simulink library "Plant"  (Simulink 7.8)
settings: Solver=ode45  StartTime=0.0  StopTime=10.0  RelTol=1e-3
undefined symbols (not defined in the file): beaver_b, beaver_c, beaver_init_p, beaver_init_pitch, beaver_init_q, beaver_init_r, beaver_init_roll, beaver_mass, Cl0, Cl_alpha2_dpt, Cl_beta, Cl_da, Cl_da_alpha, Cl_dr, Cl_p, Cl_r, Cm0, Cm_alpha, Cm_alpha2, Cm_beta2, Cm_de, Cm_df, Cm_dpt, Cm_q, Cm_r, Cn0, Cn_beta, Cn_beta3, Cn_da, Cn_dpt3, Cn_dr, Cn_p, Cn_q, Cn_r, Cx0, Cx_alpha, Cx_alpha2, Cx_alpha3, Cx_df, Cx_df_alpha, Cx_dpt, Cx_dpt2_alpha, Cx_dr, Cx_q, Cy0, Cy_beta, Cy_da, Cy_dr, Cy_dr_alpha, Cy_p, Cy_r, Cz0, Cz_alpha, Cz_alpha3, Cz_de, Cz_de_beta, Cz_df, Cz_df_alpha, Cz_dpt, Cz_q ... (+8)
libraries: aerolibconvert2 x5, aerolibasang x3, aerolibactuator x3, aerolibwind2 x3, aerolib6dof2 x1, aerolibadyn x1, aerolibatmos2 x1, aerolibobsolete x1, simulink x1
settings Model: Creator=fguerin  LastModifiedBy=fguerin

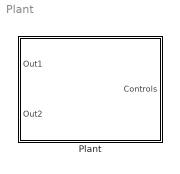
== system Plant ==
  Plant : Subsystem  TreatAsAtomicUnit=on
      mask Display: image(imread('asbbeaver.jpg'))

== system Plant/Plant ==
  Controls : Inport
  Air Data Sensor : Subsystem  TreatAsAtomicUnit=on
  DeHavilland Beaver Airframe : Subsystem
  Environment : Subsystem
  Inertial Data Sensor : Subsystem  TreatAsAtomicUnit=on
  Model Info : simulink/Model-Wide Utilities/Model Info  InitialBlockCM=None  BlockCM=None  Frame=on  DisplayStringWithTags=|  HorizontalTextAlignment=Center  LeftAlignmentValue=0.5  SourceBlockDiagram=Plant  TagMaxNumber=20
      | DeHavilland Beaver model 
      | based on original work created by
      | Marc Rauw for Delft University of Technology.  
      | http://www.dutchroll.com
  Out1 : Outport
  Out2 : Outport  Port=2
  wires:
  Controls/1 -> DeHavilland Beaver Airframe/2(Pilot)
  Air Data Sensor/1(Air Data) -> Out2/1
  Inertial Data Sensor/1(Inertial) -> Out1/1
  Environment/1(EnvBus) -> DeHavilland Beaver Airframe/1(EnvirBus)
  DeHavilland Beaver Airframe/1(ACBus) -> Environment/1(ACBus), Air Data Sensor/1(AC Bus), Inertial Data Sensor/1(AC Bus)

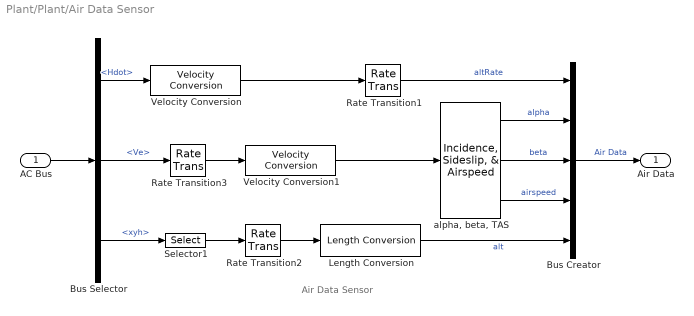
== system Plant/Plant/Air Data Sensor ==
  note: Air Data Sensor
  AC Bus : Inport
  Bus Creator : BusCreator  Inputs=5
  Bus Selector : BusSelector  OutputSignals=Hdot,Ve,xyh
  Length Conversion : aerolibconvert2/Length Conversion  IU=m  OU=ft
  Rate Transition1 : RateTransition  OutPortSampleTime=1/40
  Rate Transition2 : RateTransition  X0=2202  OutPortSampleTime=1/40
  Rate Transition3 : RateTransition  X0=[44.54 2.714 5.836]  OutPortSampleTime=1/40
  Selector1 : Selector  InputPortWidth=3  IndexOptions=Index vector (dialog)  Indices=[3]  OutputSizes=1
  Velocity Conversion : aerolibconvert2/Velocity Conversion  IU=m/s  OU=ft/s
  Velocity Conversion1 : aerolibconvert2/Velocity Conversion  IU=m/s  OU=ft/s
  "alpha, beta, TAS" : aerolibasang/Incidence, Sideslip, & Airspeed
  Air Data : Outport
  wires:
  Rate Transition2/1 -> Length Conversion/1
  Rate Transition3/1 -> Velocity Conversion1/1
  Velocity Conversion1/1 -> "alpha, beta, TAS"/1
  Length Conversion/1 -> Bus Creator/5  "alt"
  Velocity Conversion/1 -> Rate Transition1/1
  "alpha, beta, TAS"/3 -> Bus Creator/4  "airspeed"
  "alpha, beta, TAS"/2 -> Bus Creator/3  "beta"
  "alpha, beta, TAS"/1 -> Bus Creator/2  "alpha"
  Selector1/1 -> Rate Transition2/1
  Rate Transition1/1 -> Bus Creator/1  "altRate"
  Bus Creator/1 -> Air Data/1  "Air Data"
  Bus Selector/3 -> Selector1/1  "<xyh>"
  Bus Selector/2 -> Rate Transition3/1  "<Ve>"
  Bus Selector/1 -> Velocity Conversion/1  "<Hdot>"
  AC Bus/1 -> Bus Selector/1

== system Plant/Plant/DeHavilland Beaver Airframe ==
  note: DeHavilland Beaver Airframe
  EnvirBus : Inport
  Pilot : Inport  Port=2
  Aircraft Dynamics : Subsystem
  Calculate Parameters : Subsystem
  ACBus : Outport
  wires:
  Calculate Parameters/1(FltParams) -> Aircraft Dynamics/3(FltParams)
  EnvirBus/1 -> Calculate Parameters/1(EnvirBus), Aircraft Dynamics/2(EnvirBus)
  Aircraft Dynamics/1(AC Bus) -> Calculate Parameters/2(ACBus), ACBus/1
  Pilot/1 -> Aircraft Dynamics/1(Pilot)

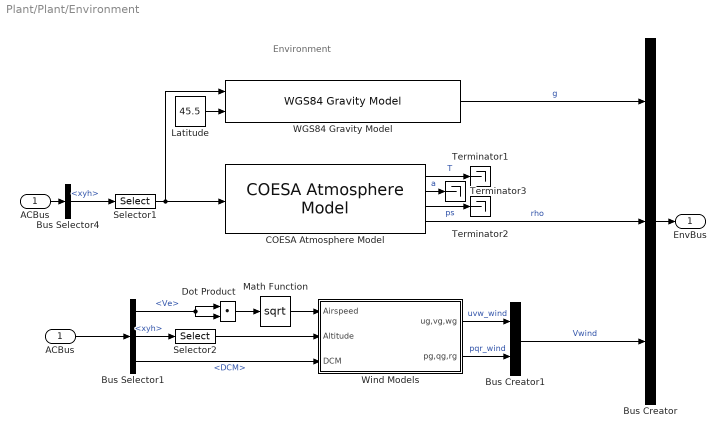
== system Plant/Plant/Environment ==
  note: Environment
  ACBus : Inport
  "ACBus " : InportShadow  Port=1
  Bus Creator : BusCreator  Inputs=3
  Bus Creator1 : BusCreator  Inputs=2
  Bus Selector1 : BusSelector  OutputSignals=Ve,xyh,DCM
  Bus Selector4 : BusSelector  OutputSignals=xyh
  COESA Atmosphere Model : aerolibatmos2/COESA Atmosphere Model  units=Metric (MKS)  spec=1976 COESA-extended U.S. Standard Atmosphere  model=Profile  profile_var=High temperature  profile_percent=1%  profile_alt=5 km (16404 ft)  envelope_var=High temperature  envelope_percent=1%  action=Warning
  Dot Product : DotProduct  InputSameDT=on  OutDataTypeStr=Inherit: Inherit via internal rule
  Latitude : Constant  Value=45.5
  Math Function : Math  Operator=sqrt  SaturateOnIntegerOverflow=on
  Selector1 : Selector  InputPortWidth=3  IndexOptions=Index vector (dialog)  Indices=[3]  OutputSizes=1
  Selector2 : Selector  InputPortWidth=3  IndexOptions=Index vector (dialog)  Indices=[3]  OutputSizes=1
  Terminator1 : Terminator
  Terminator2 : Terminator
  Terminator3 : Terminator
  WGS84 Gravity Model : aerolibobsolete/WGS84 Gravity Model  model=WGS84 Taylor Series  units=Metric (MKS)  no_atmos=on  precessing=on  month=February  day=1  year=2000  no_centrifugal=on  action=Warning
  Wind Models : Subsystem
  EnvBus : Outport
  wires:
  Bus Selector1/1 -> Dot Product/2, Dot Product/1  "<Ve>"
  Selector2/1 -> Wind Models/2(Altitude)
  Bus Selector1/2 -> Selector2/1  "<xyh>"
  "ACBus "/1 -> Bus Selector1/1
  Bus Selector4/1 -> Selector1/1  "<xyh>"
  ACBus/1 -> Bus Selector4/1
  Bus Creator/1 -> EnvBus/1
  Math Function/1 -> Wind Models/1(Airspeed)
  Dot Product/1 -> Math Function/1
  Bus Creator1/1 -> Bus Creator/3  "Vwind"
  Wind Models/1(ug,vg,wg) -> Bus Creator1/1  "uvw_wind"
  Wind Models/2(pg,qg,rg) -> Bus Creator1/2  "pqr_wind"
  Bus Selector1/3 -> Wind Models/3(DCM)  "<DCM>"
  WGS84 Gravity Model/1 -> Bus Creator/1  "g"
  Latitude/1 -> WGS84 Gravity Model/2
  Selector1/1 -> WGS84 Gravity Model/1, COESA Atmosphere Model/1
  COESA Atmosphere Model/2 -> Terminator3/1  "a"
  COESA Atmosphere Model/3 -> Terminator2/1  "ps"
  COESA Atmosphere Model/1 -> Terminator1/1  "T"
  COESA Atmosphere Model/4 -> Bus Creator/2  "rho"

== system Plant/Plant/Inertial Data Sensor ==
  note: Inertial Data Sensor
  AC Bus : Inport
  Angle Conversion3 : aerolibconvert2/Angle Conversion  IU=rad  OU=deg
  Angle Conversion5 : aerolibconvert2/Angle Conversion  IU=rad  OU=deg
  Bus Creator : BusCreator  Inputs=6
  Bus Selector : BusSelector  OutputSignals=phi_theta_psi,pqr
  Demux : Demux  Outputs=3
  Demux1 : Demux  Outputs=3
  Rate Transition1 : RateTransition  X0=beaver_init_roll/pi*180  OutPortSampleTime=1/40
  Rate Transition2 : RateTransition  X0=beaver_init_pitch/pi*180  OutPortSampleTime=1/40
  Rate Transition3 : RateTransition  X0=heading0  OutPortSampleTime=1/40
  Rate Transition4 : RateTransition  OutPortSampleTime=1/40
  Inertial : Outport
  wires:
  Angle Conversion5/1 -> Demux1/1
  Demux1/3 -> Rate Transition3/1
  Demux1/2 -> Rate Transition2/1
  Demux1/1 -> Rate Transition1/1
  Bus Selector/1 -> Angle Conversion5/1  "<phi_theta_psi>"
  Angle Conversion3/1 -> Rate Transition4/1
  Rate Transition4/1 -> Demux/1
  Rate Transition3/1 -> Bus Creator/3  "psi"
  Rate Transition2/1 -> Bus Creator/2  "theta"
  Rate Transition1/1 -> Bus Creator/1  "phi"
  Demux/1 -> Bus Creator/4  "p"
  Demux/3 -> Bus Creator/6  "r"
  Bus Creator/1 -> Inertial/1  "Inertial"
  Demux/2 -> Bus Creator/5  "q"
  Bus Selector/2 -> Angle Conversion3/1  "<pqr>"
  AC Bus/1 -> Bus Selector/1

== system Plant/Plant/DeHavilland Beaver Airframe/Aircraft Dynamics ==
  Pilot : Inport
  EnvirBus : Inport  Port=2
  FltParams : Inport  Port=3
  6DoF (Quaternion) : aerolib6dof2/6DoF (Euler Angles)  units=Metric (MKS)  mtype=Fixed  rep=Quaternion  xme_0=xme_0  Vm_0=[44.54 2.714 5.836]  eul_0=[beaver_init_roll, beaver_init_pitch, heading0/180*pi]  pm_0=[beaver_init_p, beaver_init_q, beaver_init_r]  mass_0=beaver_mass  mass_e=0  mass_f=0  inertia="[5.787969e3  0 1.1764e2; 0 6.92893e3 0; -1.1764e2 0 1.1578329e4]"  inertia_e=eye(3)  inertia_f=eye(3)  k_quat=1.0
  Bus Creator : BusCreator  Inputs=8
  Hdot : Gain  Gain=-1  SaturateOnIntegerOverflow=on  OutDataTypeStr=Inherit: Same as input  ParamDataTypeStr=Inherit: Same as input
  Selector1 : Selector  InputPortWidth=3  IndexOptions=Index vector (dialog)  Indices=[3]  OutputSizes=1
  Terminator : Terminator
  Terminator1 : Terminator
  Total Forces  and Moments : Subsystem
  xyH : Gain  Gain=[1 1 -1]  SaturateOnIntegerOverflow=on  OutDataTypeStr=Inherit: Same as input  ParamDataTypeStr=Inherit: Same as input
  AC Bus : Outport
  wires:
  FltParams/1 -> Total Forces  and Moments/4(FltParams)
  6DoF (Quaternion)/6 -> Bus Creator/8  "pqr"
  EnvirBus/1 -> Total Forces  and Moments/1(EnvirBus)
  Bus Creator/1 -> AC Bus/1
  6DoF (Quaternion)/8 -> Terminator1/1
  Hdot/1 -> Bus Creator/1  "Hdot"
  xyH/1 -> Bus Creator/4  "xyh"
  Total Forces  and Moments/2(Total Moment) -> 6DoF (Quaternion)/2
  Total Forces  and Moments/1(Total Force) -> 6DoF (Quaternion)/1
  Selector1/1 -> Hdot/1
  Pilot/1 -> Total Forces  and Moments/2(Pilot)
  6DoF (Quaternion)/1 -> Bus Creator/2, Selector1/1  "Ve"
  6DoF (Quaternion)/7 -> Terminator/1
  6DoF (Quaternion)/5 -> Bus Creator/7  "Vbody"
  6DoF (Quaternion)/2 -> Bus Creator/3, xyH/1  "Xe"
  6DoF (Quaternion)/3 -> Bus Creator/5  "phi_theta_psi"
  6DoF (Quaternion)/4 -> Total Forces  and Moments/3(DCM), Bus Creator/6  "DCM"

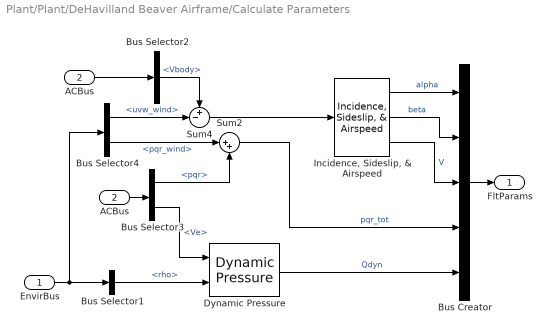
== system Plant/Plant/DeHavilland Beaver Airframe/Calculate Parameters ==
  EnvirBus : Inport
  ACBus : Inport  Port=2
  "ACBus " : InportShadow  Port=2
  Bus Creator : BusCreator  Inputs=5
  Bus Selector1 : BusSelector  OutputSignals=rho
  Bus Selector2 : BusSelector  OutputSignals=Vbody
  Bus Selector3 : BusSelector  OutputSignals=pqr,Ve
  Bus Selector4 : BusSelector  OutputSignals=Vwind.uvw_wind,Vwind.pqr_wind
  Dynamic Pressure : aerolibasang/Dynamic Pressure
  "Incidence, Sideslip, & Airspeed" : aerolibasang/Incidence, Sideslip, & Airspeed
  Sum2 : Sum  Inputs=|++  SaturateOnIntegerOverflow=on  InputSameDT=on  OutDataTypeStr=Inherit: Same as first input
  Sum4 : Sum  Inputs=+-|  SaturateOnIntegerOverflow=on  InputSameDT=on  OutDataTypeStr=Inherit: Same as first input
  FltParams : Outport
  wires:
  Sum2/1 -> Bus Creator/4  "pqr_tot"
  Bus Selector4/1 -> Sum4/2  "<uvw_wind>"
  Bus Selector2/1 -> Sum4/1  "<Vbody>"
  "Incidence, Sideslip, & Airspeed"/3 -> Bus Creator/3  "V"
  "Incidence, Sideslip, & Airspeed"/2 -> Bus Creator/2  "beta"
  "Incidence, Sideslip, & Airspeed"/1 -> Bus Creator/1  "alpha"
  Sum4/1 -> "Incidence, Sideslip, & Airspeed"/1
  Bus Selector4/2 -> Sum2/1  "<pqr_wind>"
  Bus Selector3/2 -> Dynamic Pressure/1  "<Ve>"
  Dynamic Pressure/1 -> Bus Creator/5  "Qdyn"
  EnvirBus/1 -> Bus Selector4/1, Bus Selector1/1
  Bus Selector1/1 -> Dynamic Pressure/2  "<rho>"
  ACBus/1 -> Bus Selector3/1
  Bus Selector3/1 -> Sum2/2  "<pqr>"
  Bus Creator/1 -> FltParams/1
  "ACBus "/1 -> Bus Selector2/1

== system Plant/Plant/Environment/Wind Models ==
  Airspeed : Inport
  Altitude : Inport  Port=2
  DCM : Inport  Port=3
  "DCM " : InportShadow  Port=3
  Discrete Wind Gust Model : aerolibwind2/Discrete Wind Gust Model  units=Metric (MKS)  Gx=off  Gy=off  Gz=off  t_0=20  d_m=[120 120 80]  v_m=[3.5 3.5 3.0]
  Dryden Wind Turbulence Model  (Continuous (+q -r)) : aerolibwind2/Dryden Wind Turbulence Model  (Continuous (+q -r))  units=Metric (MKS)  spec=MIL-F-8785C  model=Continuous Dryden (+q -r)  W20=5  Wdeg=0  TurbProb=10^-2 - Light  L_high=533.4  Wingspan=4  ts=0.1  Seed=[23341 23342 23343 23344]  T_on=off
  Sum : Sum  Inputs=+++  SaturateOnIntegerOverflow=on  InputSameDT=on  OutDataTypeStr=Inherit: Same as first input
  Wind Shear Model : aerolibwind2/Wind Shear Model  units=Metric (MKS)  phase=Category C - Terminal Flight Phase  W_20=0  Wdeg=0
  ug,vg,wg : Outport
  pg,qg,rg : Outport  Port=2
  wires:
  Altitude/1 -> Wind Shear Model/1, Dryden Wind Turbulence Model  (Continuous (+q -r))/1
  Dryden Wind Turbulence Model  (Continuous (+q -r))/2 -> pg,qg,rg/1
  Airspeed/1 -> Discrete Wind Gust Model/1, Dryden Wind Turbulence Model  (Continuous (+q -r))/2
  DCM/1 -> Wind Shear Model/2
  Sum/1 -> ug,vg,wg/1
  Discrete Wind Gust Model/1 -> Sum/3
  Dryden Wind Turbulence Model  (Continuous (+q -r))/1 -> Sum/2
  Wind Shear Model/1 -> Sum/1
  "DCM "/1 -> Dryden Wind Turbulence Model  (Continuous (+q -r))/3

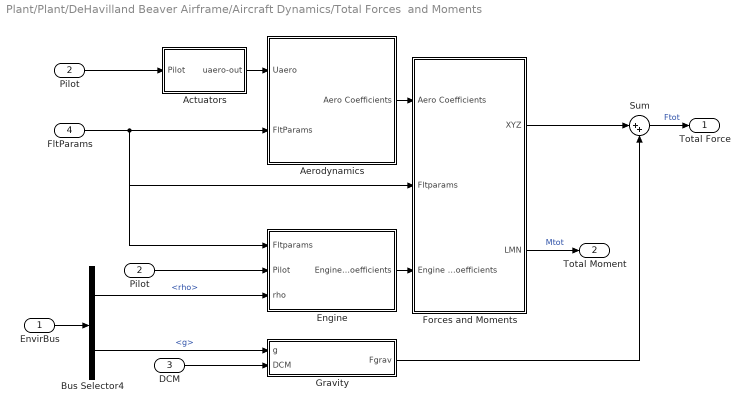
== system Plant/Plant/DeHavilland Beaver Airframe/Aircraft Dynamics/Total Forces  and Moments ==
  EnvirBus : Inport
  Pilot : Inport  Port=2
  DCM : Inport  Port=3
  FltParams : Inport  Port=4
  Actuators : Subsystem
  Aerodynamics : Subsystem
  Bus Selector4 : BusSelector  OutputSignals=rho,g
  "Engine " : Subsystem
  Forces and Moments : Subsystem
  "Gravity " : Subsystem
  "Pilot " : InportShadow  Port=2
  Sum : Sum  Inputs=|++  SaturateOnIntegerOverflow=on  InputSameDT=on  OutDataTypeStr=Inherit: Same as first input
  Total Force : Outport
  Total Moment : Outport  Port=2
  wires:
  EnvirBus/1 -> Bus Selector4/1
  Actuators/1(uaero-out) -> Aerodynamics/1(Uaero)
  FltParams/1 -> Aerodynamics/2(FltParams), Forces and Moments/2(Fltparams), "Engine "/1(Fltparams)
  "Pilot "/1 -> "Engine "/2(Pilot)
  Forces and Moments/2(LMN) -> Total Moment/1  "Mtot"
  Sum/1 -> Total Force/1  "Ftot"
  Bus Selector4/2 -> "Gravity "/1(g)  "<g>"
  DCM/1 -> "Gravity "/2(DCM)
  Bus Selector4/1 -> "Engine "/3(rho)  "<rho>"
  Pilot/1 -> Actuators/1(Pilot)
  Aerodynamics/1(Aero Coefficients) -> Forces and Moments/1(Aero Coefficients)
  "Gravity "/1(Fgrav) -> Sum/2
  "Engine "/1(Engine Coefficients) -> Forces and Moments/3(Engine Coefficients)
  Forces and Moments/1(XYZ) -> Sum/1

== system Plant/Plant/DeHavilland Beaver Airframe/Aircraft Dynamics/Total Forces  and Moments/Actuators ==
  Pilot : Inport
  Aileron Actuator : aerolibactuator/Second Order Nonlinear Actuator  wn_fin=10*2*pi  z_fin=0.7  fin_max=15*pi/180  fin_min=-15*pi/180  fin_maxrate=40*pi/180  fin_act_0=uaero0(3)
  Bus Selector2 : BusSelector  OutputSignals=uaero
  Demux : Demux
  Elevator Actuator : aerolibactuator/Second Order Nonlinear Actuator  wn_fin=10*2*pi  z_fin=0.7  fin_max=20*pi/180  fin_min=-20*pi/180  fin_maxrate=40*pi/180  fin_act_0=uaero0(1)
  Initial inputs for aero : Constant  Value=uaero0
  Mux : Mux
  Rudder Actuator : aerolibactuator/Second Order Nonlinear Actuator  wn_fin=10*2*pi  z_fin=0.7  fin_max=25*pi/180  fin_min=-25*pi/180  fin_maxrate=40*pi/180  fin_act_0=uaero0(3)
  Sum1 : Sum  Inputs=++|  SaturateOnIntegerOverflow=on  InputSameDT=on  OutDataTypeStr=Inherit: Same as first input
  uaero-out : Outport
  wires:
  Rudder Actuator/1 -> Mux/3
  Aileron Actuator/1 -> Mux/2
  Elevator Actuator/1 -> Mux/1
  Bus Selector2/1 -> Sum1/2  "<uaero>"
  Sum1/1 -> Demux/1
  Mux/1 -> uaero-out/1
  Demux/3 -> Rudder Actuator/1
  Demux/2 -> Aileron Actuator/1
  Demux/1 -> Elevator Actuator/1
  Demux/4 -> Mux/4
  Initial inputs for aero/1 -> Sum1/1
  Pilot/1 -> Bus Selector2/1

== system Plant/Plant/DeHavilland Beaver Airframe/Aircraft Dynamics/Total Forces  and Moments/Aerodynamics ==
  Uaero : Inport
  FltParams : Inport  Port=2
  Actuator Increments : Subsystem
  Body Rate Damping : Subsystem
  Bus Selector1 : BusSelector  OutputSignals=alpha,beta
  Bus Selector2 : BusSelector  OutputSignals=V,pqr_tot
  Datum Coefficients : Subsystem
  Sum : Sum  Inputs=+++  SaturateOnIntegerOverflow=on
  Aero Coefficients : Outport
  wires:
  FltParams/1 -> Bus Selector2/1, Bus Selector1/1
  Bus Selector1/1 -> Datum Coefficients/1(alpha), Actuator Increments/1(alpha)  "<alpha>"
  Uaero/1 -> Actuator Increments/3(Actuator Deflections)
  Bus Selector2/2 -> Body Rate Damping/2(p,q,r)  "<pqr_tot>"
  Bus Selector2/1 -> Body Rate Damping/1(V)  "<V>"
  Actuator Increments/1(Coefficients) -> Sum/2
  Datum Coefficients/1(Coefficients) -> Sum/1
  Body Rate Damping/1(Coefficients) -> Sum/3
  Sum/1 -> Aero Coefficients/1
  Bus Selector1/2 -> Datum Coefficients/2(beta), Actuator Increments/2(beta)  "<beta>"

== system Plant/Plant/DeHavilland Beaver Airframe/Aircraft Dynamics/Total Forces  and Moments/Engine  ==
  Fltparams : Inport
  Pilot : Inport  Port=2
  rho : Inport  Port=3
  Bus Selector4 : BusSelector  OutputSignals=V,alpha
  eng : Subsystem
  pow : Subsystem
  Engine Coefficients : Outport
  wires:
  Fltparams/1 -> Bus Selector4/1
  pow/1(dpt) -> eng/1(dpt)
  Pilot/1 -> pow/2(Pilot)
  eng/1(Cprop) -> Engine Coefficients/1
  Bus Selector4/2 -> eng/2(alpha)  "<alpha>"
  rho/1 -> pow/1(rho)
  Bus Selector4/1 -> pow/3(V)  "<V>"

== system Plant/Plant/DeHavilland Beaver Airframe/Aircraft Dynamics/Total Forces  and Moments/Forces and Moments ==
  Aero Coefficients : Inport
  Fltparams : Inport  Port=2
  Engine Coefficients : Inport  Port=3
  Aerodynamic Forces and Moments : aerolibadyn/Aerodynamic Forces and Moments   inputAxes=Body  outputForceAxes=Body  outputMomentAxes=Body  S=beaver_S  b=beaver_b  cbar=beaver_c
  Bus Selector4 : BusSelector  OutputSignals=Qdyn
  Sum : Sum  Inputs=++|  SaturateOnIntegerOverflow=on  InputSameDT=on  OutDataTypeStr=Inherit: Same as first input
  neglect center of gravity  and center of pressure effects : Constant  Value=[0 0 0]
  XYZ : Outport
  LMN : Outport  Port=2
  wires:
  Bus Selector4/1 -> Aerodynamic Forces and Moments/2  "<Qdyn>"
  neglect center of gravity  and center of pressure effects/1 -> Aerodynamic Forces and Moments/4, Aerodynamic Forces and Moments/3
  Aerodynamic Forces and Moments/1 -> XYZ/1
  Fltparams/1 -> Bus Selector4/1
  Aerodynamic Forces and Moments/2 -> LMN/1
  Engine Coefficients/1 -> Sum/1
  Aero Coefficients/1 -> Sum/2
  Sum/1 -> Aerodynamic Forces and Moments/1

== system Plant/Plant/DeHavilland Beaver Airframe/Aircraft Dynamics/Total Forces  and Moments/Gravity  ==
  g : Inport
  DCM : Inport  Port=2
  Gravity in Earth Axes : Gain  Gain=[0 0 beaver_mass]  SaturateOnIntegerOverflow=on  OutDataTypeStr=Inherit: Same as input  ParamDataTypeStr=Inherit: Same as input
  Inertial to Body : Product  Multiplication=Matrix(*)  SaturateOnIntegerOverflow=on  InputSameDT=on  OutDataTypeStr=Inherit: Same as first input
  Reshape : Reshape  OutputDimensionality=Column vector (2-D)
  Reshape1 : Reshape
  Fgrav : Outport
  wires:
  Reshape1/1 -> Fgrav/1
  Reshape/1 -> Inertial to Body/2
  Gravity in Earth Axes/1 -> Reshape/1
  DCM/1 -> Inertial to Body/1
  g/1 -> Gravity in Earth Axes/1
  Inertial to Body/1 -> Reshape1/1

== system Plant/Plant/DeHavilland Beaver Airframe/Aircraft Dynamics/Total Forces  and Moments/Aerodynamics/Actuator Increments ==
  alpha : Inport
  beta : Inport  Port=2
  Actuator Deflections : Inport  Port=3
  Aileron : Subsystem  AncestorBlock=|
      | aeroblk_lib_HL20/HL20
      | Airframe/Aerodynamic
      | Coefficients/Actuator
      | Increments/Aileron
  Elevator : Subsystem  AncestorBlock=|
      | aeroblk_lib_HL20/HL20
      | Airframe/Aerodynamic
      | Coefficients/Actuator
      | Increments/Elevator
  Flap : Subsystem  AncestorBlock=|
      | aeroblk_lib_HL20/HL20
      | Airframe/Aerodynamic
      | Coefficients/Actuator
      | Increments/Flap(pos)
  Rudder : Subsystem  AncestorBlock=|
      | aeroblk_lib_HL20/HL20
      | Airframe/Aerodynamic
      | Coefficients/Actuator
      | Increments/Rudder
  Sum : Sum  Inputs=++++  SaturateOnIntegerOverflow=on  InputSameDT=on  OutDataTypeStr=Inherit: Same as first input
  Coefficients : Outport
  wires:
  Sum/1 -> Coefficients/1
  Flap/1(delCoeff) -> Sum/4
  Rudder/1(delCoeff) -> Sum/3
  Elevator/1(delCoeff) -> Sum/2
  Aileron/1(delCoeff) -> Sum/1
  beta/1 -> Elevator/2(Beta)
  alpha/1 -> Aileron/1(alpha), Rudder/1(Alpha), Flap/1(Alpha)
  Actuator Deflections/1 -> Rudder/2(Actuators), Elevator/1(Actuators), Aileron/2(Actuators), Flap/2(Actuators)

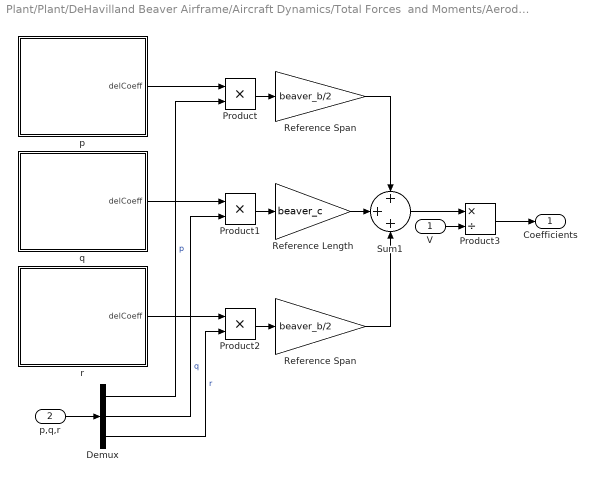
== system Plant/Plant/DeHavilland Beaver Airframe/Aircraft Dynamics/Total Forces  and Moments/Aerodynamics/Body Rate Damping ==
  V : Inport
  p,q,r : Inport  Port=2
  Demux : Demux  Outputs=3
  Product : Product  SaturateOnIntegerOverflow=on  InputSameDT=on  OutDataTypeStr=Inherit: Same as first input
  Product1 : Product  SaturateOnIntegerOverflow=on  InputSameDT=on  OutDataTypeStr=Inherit: Same as first input
  Product2 : Product  SaturateOnIntegerOverflow=on  InputSameDT=on  OutDataTypeStr=Inherit: Same as first input
  Product3 : Product  Inputs=*/  SaturateOnIntegerOverflow=on  InputSameDT=on  OutDataTypeStr=Inherit: Same as first input
  Reference Length : Gain  Gain=beaver_c  SaturateOnIntegerOverflow=on  OutDataTypeStr=Inherit: Same as input  ParamDataTypeStr=Inherit: Same as input
  Reference Span : Gain  Gain=beaver_b/2  SaturateOnIntegerOverflow=on  OutDataTypeStr=Inherit: Same as input  ParamDataTypeStr=Inherit: Same as input
  "Reference Span " : Gain  Gain=beaver_b/2  SaturateOnIntegerOverflow=on  OutDataTypeStr=Inherit: Same as input  ParamDataTypeStr=Inherit: Same as input
  Sum1 : Sum  Inputs=+++  SaturateOnIntegerOverflow=on  InputSameDT=on  OutDataTypeStr=Inherit: Same as first input
  p : Subsystem
  q : Subsystem
  r : Subsystem
  Coefficients : Outport
  wires:
  "Reference Span "/1 -> Sum1/3
  Reference Span/1 -> Sum1/1
  Reference Length/1 -> Sum1/2
  r/1(delCoeff) -> Product2/1
  Product/1 -> Reference Span/1
  Product2/1 -> "Reference Span "/1
  Product1/1 -> Reference Length/1
  Product3/1 -> Coefficients/1
  V/1 -> Product3/2
  Sum1/1 -> Product3/1
  Demux/3 -> Product2/2  "r"
  Demux/2 -> Product1/2  "q"
  Demux/1 -> Product/2  "p"
  p,q,r/1 -> Demux/1
  q/1(delCoeff) -> Product1/1
  p/1(delCoeff) -> Product/1

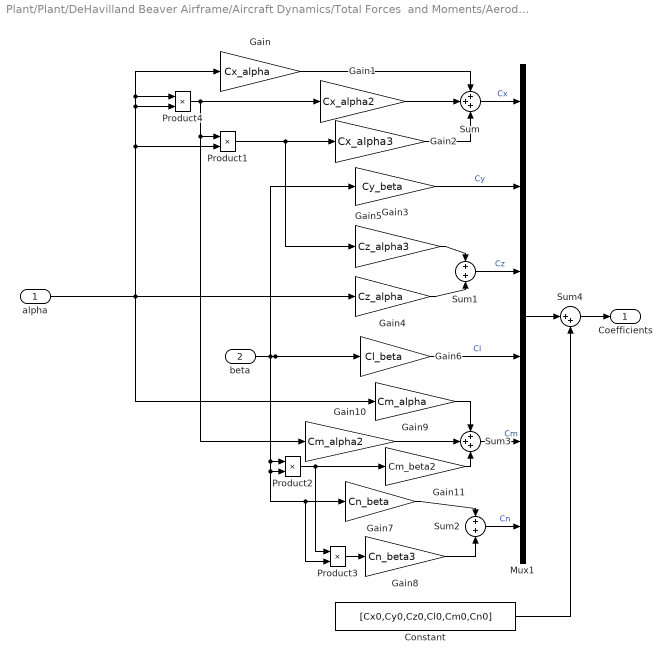
== system Plant/Plant/DeHavilland Beaver Airframe/Aircraft Dynamics/Total Forces  and Moments/Aerodynamics/Datum Coefficients ==
  alpha : Inport
  beta : Inport  Port=2
  Constant : Constant  Value=[Cx0,Cy0,Cz0,Cl0,Cm0,Cn0]
  Gain : Gain  Gain=Cx_alpha  SaturateOnIntegerOverflow=on  OutDataTypeStr=Inherit: Same as input  ParamDataTypeStr=Inherit: Same as input
  Gain1 : Gain  Gain=Cx_alpha2  SaturateOnIntegerOverflow=on  OutDataTypeStr=Inherit: Same as input  ParamDataTypeStr=Inherit: Same as input
  Gain10 : Gain  Gain=Cm_alpha2  SaturateOnIntegerOverflow=on  OutDataTypeStr=Inherit: Same as input  ParamDataTypeStr=Inherit: Same as input
  Gain11 : Gain  Gain=Cm_beta2  SaturateOnIntegerOverflow=on  OutDataTypeStr=Inherit: Same as input  ParamDataTypeStr=Inherit: Same as input
  Gain2 : Gain  Gain=Cx_alpha3  SaturateOnIntegerOverflow=on  OutDataTypeStr=Inherit: Same as input  ParamDataTypeStr=Inherit: Same as input
  Gain3 : Gain  Gain=Cy_beta  SaturateOnIntegerOverflow=on  OutDataTypeStr=Inherit: Same as input  ParamDataTypeStr=Inherit: Same as input
  Gain4 : Gain  Gain=Cz_alpha  SaturateOnIntegerOverflow=on  OutDataTypeStr=Inherit: Same as input  ParamDataTypeStr=Inherit: Same as input
  Gain5 : Gain  Gain=Cz_alpha3  SaturateOnIntegerOverflow=on  OutDataTypeStr=Inherit: Same as input  ParamDataTypeStr=Inherit: Same as input
  Gain6 : Gain  Gain=Cl_beta  SaturateOnIntegerOverflow=on  OutDataTypeStr=Inherit: Same as input  ParamDataTypeStr=Inherit: Same as input
  Gain7 : Gain  Gain=Cn_beta  SaturateOnIntegerOverflow=on  OutDataTypeStr=Inherit: Same as input  ParamDataTypeStr=Inherit: Same as input
  Gain8 : Gain  Gain=Cn_beta3  SaturateOnIntegerOverflow=on  OutDataTypeStr=Inherit: Same as input  ParamDataTypeStr=Inherit: Same as input
  Gain9 : Gain  Gain=Cm_alpha  SaturateOnIntegerOverflow=on  OutDataTypeStr=Inherit: Same as input  ParamDataTypeStr=Inherit: Same as input
  Mux1 : Mux  Inputs=6
  Product{1..4} (4 alike) : Product  SaturateOnIntegerOverflow=on  InputSameDT=on  OutDataTypeStr=Inherit: Same as first input
  Sum : Sum  Inputs=+++  SaturateOnIntegerOverflow=on
  Sum1 : Sum  SaturateOnIntegerOverflow=on
  Sum2 : Sum  SaturateOnIntegerOverflow=on
  Sum3 : Sum  Inputs=+++  SaturateOnIntegerOverflow=on
  Sum4 : Sum  Inputs=|++  SaturateOnIntegerOverflow=on
  Coefficients : Outport
  wires:
  beta/1 -> Gain6/1, Product2/1, Product2/2, Gain7/1, Product3/2, Gain3/1
  alpha/1 -> Gain4/1, Gain9/1, Gain/1, Product4/1, Product4/2, Product1/2
  Gain6/1 -> Mux1/4  "Cl"
  Gain3/1 -> Mux1/2  "Cy"
  Sum1/1 -> Mux1/3  "Cz"
  Sum/1 -> Mux1/1  "Cx"
  Sum2/1 -> Mux1/6  "Cn"
  Gain/1 -> Sum/1
  Gain1/1 -> Sum/2
  Product4/1 -> Gain1/1, Gain10/1, Product1/1
  Gain2/1 -> Sum/3
  Product1/1 -> Gain2/1, Gain5/1
  Gain4/1 -> Sum1/2
  Gain5/1 -> Sum1/1
  Gain7/1 -> Sum2/1
  Gain8/1 -> Sum2/2
  Product3/1 -> Gain8/1
  Sum3/1 -> Mux1/5  "Cm"
  Gain9/1 -> Sum3/1
  Gain11/1 -> Sum3/3
  Product2/1 -> Gain11/1, Product3/1
  Gain10/1 -> Sum3/2
  Mux1/1 -> Sum4/1
  Sum4/1 -> Coefficients/1
  Constant/1 -> Sum4/2

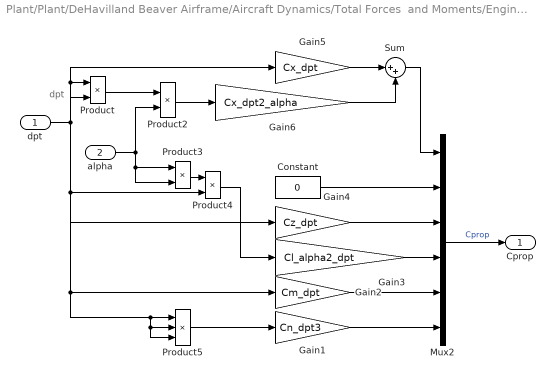
== system Plant/Plant/DeHavilland Beaver Airframe/Aircraft Dynamics/Total Forces  and Moments/Engine /eng ==
  note: dpt
  dpt : Inport
  alpha : Inport  Port=2
  Constant : Constant  Value=0
  Gain1 : Gain  Gain=Cn_dpt3  SaturateOnIntegerOverflow=on  OutDataTypeStr=Inherit: Same as input  ParamDataTypeStr=Inherit: Same as input
  Gain2 : Gain  Gain=Cm_dpt  SaturateOnIntegerOverflow=on  OutDataTypeStr=Inherit: Same as input  ParamDataTypeStr=Inherit: Same as input
  Gain3 : Gain  Gain=Cl_alpha2_dpt  SaturateOnIntegerOverflow=on  OutDataTypeStr=Inherit: Same as input  ParamDataTypeStr=Inherit: Same as input
  Gain4 : Gain  Gain=Cz_dpt  SaturateOnIntegerOverflow=on  OutDataTypeStr=Inherit: Same as input  ParamDataTypeStr=Inherit: Same as input
  Gain5 : Gain  Gain=Cx_dpt  SaturateOnIntegerOverflow=on  OutDataTypeStr=Inherit: Same as input  ParamDataTypeStr=Inherit: Same as input
  Gain6 : Gain  Gain=Cx_dpt2_alpha  SaturateOnIntegerOverflow=on  OutDataTypeStr=Inherit: Same as input  ParamDataTypeStr=Inherit: Same as input
  Mux2 : Mux  Inputs=6
  Product{,2..4} (4 alike) : Product  SaturateOnIntegerOverflow=on  OutDataTypeStr=Inherit: Same as first input
  Product5 : Product  Inputs=3  SaturateOnIntegerOverflow=on  OutDataTypeStr=Inherit: Same as first input
  Sum : Sum  Inputs=|++  SaturateOnIntegerOverflow=on
  Cprop : Outport
  wires:
  Product3/1 -> Product4/1
  Product/1 -> Product2/1
  Mux2/1 -> Cprop/1  "Cprop"
  alpha/1 -> Product3/2, Product3/1, Product2/2
  dpt/1 -> Product4/2, Product/1, Product/2, Gain4/1, Gain2/1, Product5/1, Product5/2, Product5/3, Gain5/1
  Product2/1 -> Gain6/1
  Product4/1 -> Gain3/1
  Gain1/1 -> Mux2/6
  Gain2/1 -> Mux2/5
  Gain3/1 -> Mux2/4
  Gain4/1 -> Mux2/3
  Constant/1 -> Mux2/2
  Gain5/1 -> Sum/1
  Gain6/1 -> Sum/2
  Sum/1 -> Mux2/1
  Product5/1 -> Gain1/1

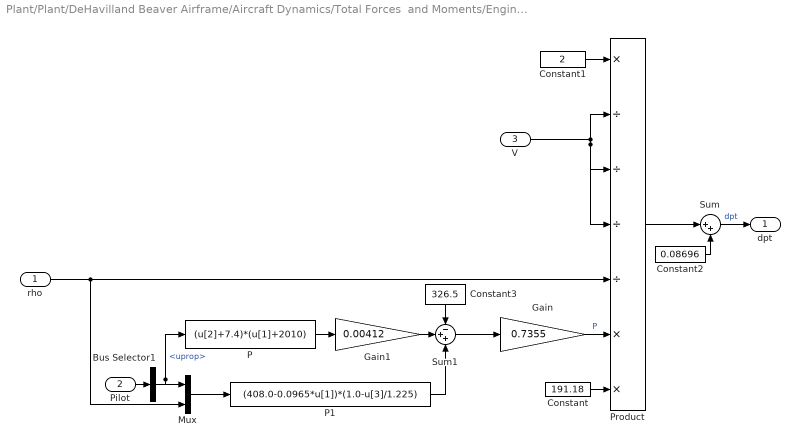
== system Plant/Plant/DeHavilland Beaver Airframe/Aircraft Dynamics/Total Forces  and Moments/Engine /pow ==
  rho : Inport
  Pilot : Inport  Port=2
  V : Inport  Port=3
  Bus Selector1 : BusSelector  OutputSignals=uprop
  Constant : Constant  Value=191.18
  Constant1 : Constant  Value=2
  Constant2 : Constant  Value=0.08696
  Constant3 : Constant  Value=326.5
  Gain : Gain  Gain=0.7355  SaturateOnIntegerOverflow=on  OutDataTypeStr=Inherit: Same as input  ParamDataTypeStr=Inherit: Same as input
  Gain1 : Gain  Gain=0.00412  SaturateOnIntegerOverflow=on  OutDataTypeStr=Inherit: Same as input  ParamDataTypeStr=Inherit: Same as input
  Mux : Mux  Inputs=2
  P : Fcn  Expr=(u[2]+7.4)*(u[1]+2010)
  P1 : Fcn  Expr=(408.0-0.0965*u[1])*(1.0-u[3]/1.225)
  Product : Product  Inputs=*////**  SaturateOnIntegerOverflow=on  OutDataTypeStr=Inherit: Same as first input
  Sum : Sum  Inputs=|++  SaturateOnIntegerOverflow=on
  Sum1 : Sum  Inputs=-++  SaturateOnIntegerOverflow=on
  dpt : Outport
  wires:
  Pilot/1 -> Bus Selector1/1
  Constant2/1 -> Sum/2
  Product/1 -> Sum/1
  Constant1/1 -> Product/1
  Constant/1 -> Product/7
  Bus Selector1/1 -> P/1, Mux/1  "<uprop>"
  V/1 -> Product/2, Product/3, Product/4
  Sum/1 -> dpt/1  "dpt"
  rho/1 -> Product/5, Mux/2
  Gain/1 -> Product/6  "P"
  P/1 -> Gain1/1
  Sum1/1 -> Gain/1
  Mux/1 -> P1/1
  Gain1/1 -> Sum1/2
  Constant3/1 -> Sum1/1
  P1/1 -> Sum1/3

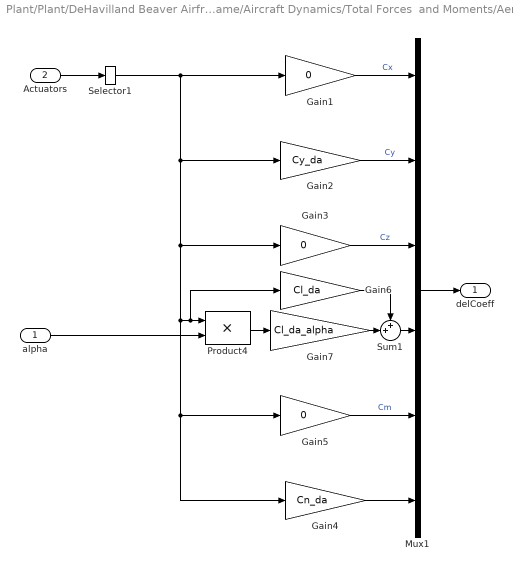
== system Plant/Plant/DeHavilland Beaver Airframe/Aircraft Dynamics/Total Forces  and Moments/Aerodynamics/Actuator Increments/Aileron ==
  alpha : Inport
  Actuators : Inport  Port=2
  Gain1 : Gain  Gain=0  SaturateOnIntegerOverflow=on  OutDataTypeStr=Inherit: Same as input  ParamDataTypeStr=Inherit: Same as input
  Gain2 : Gain  Gain=Cy_da  SaturateOnIntegerOverflow=on  OutDataTypeStr=Inherit: Same as input  ParamDataTypeStr=Inherit: Same as input
  Gain3 : Gain  Gain=0  SaturateOnIntegerOverflow=on  OutDataTypeStr=Inherit: Same as input  ParamDataTypeStr=Inherit: Same as input
  Gain4 : Gain  Gain=Cn_da  SaturateOnIntegerOverflow=on  OutDataTypeStr=Inherit: Same as input  ParamDataTypeStr=Inherit: Same as input
  Gain5 : Gain  Gain=0  SaturateOnIntegerOverflow=on  OutDataTypeStr=Inherit: Same as input  ParamDataTypeStr=Inherit: Same as input
  Gain6 : Gain  Gain=Cl_da  SaturateOnIntegerOverflow=on  OutDataTypeStr=Inherit: Same as input  ParamDataTypeStr=Inherit: Same as input
  Gain7 : Gain  Gain=Cl_da_alpha  SaturateOnIntegerOverflow=on  OutDataTypeStr=Inherit: Same as input  ParamDataTypeStr=Inherit: Same as input
  Mux1 : Mux  Inputs=6
  Product4 : Product  SaturateOnIntegerOverflow=on  InputSameDT=on  OutDataTypeStr=Inherit: Same as first input
  Selector1 : Selector  InputPortWidth=4  IndexOptions=Index vector (dialog)  Indices=2  OutputSizes=1
  Sum1 : Sum  Inputs=++|  SaturateOnIntegerOverflow=on
  delCoeff : Outport
  wires:
  Selector1/1 -> Gain4/1, Gain5/1, Product4/1, Gain6/1, Gain3/1, Gain2/1, Gain1/1
  Gain4/1 -> Mux1/6
  Gain5/1 -> Mux1/5  "Cm"
  Gain3/1 -> Mux1/3  "Cz"
  Gain2/1 -> Mux1/2  "Cy"
  Mux1/1 -> delCoeff/1
  Actuators/1 -> Selector1/1
  alpha/1 -> Product4/2
  Gain1/1 -> Mux1/1  "Cx"
  Product4/1 -> Gain7/1
  Gain7/1 -> Sum1/2
  Sum1/1 -> Mux1/4
  Gain6/1 -> Sum1/1

== system Plant/Plant/DeHavilland Beaver Airframe/Aircraft Dynamics/Total Forces  and Moments/Aerodynamics/Actuator Increments/Elevator ==
  Actuators : Inport
  Beta : Inport  Port=2
  Constant1 : Constant  Value=0
  Gain1 : Gain  Gain=Cz_de  SaturateOnIntegerOverflow=on  OutDataTypeStr=Inherit: Same as input  ParamDataTypeStr=Inherit: Same as input
  Gain2 : Gain  Gain=Cz_de_beta  SaturateOnIntegerOverflow=on  OutDataTypeStr=Inherit: Same as input  ParamDataTypeStr=Inherit: Same as input
  Gain3 : Gain  Gain=Cm_de  SaturateOnIntegerOverflow=on  OutDataTypeStr=Inherit: Same as input  ParamDataTypeStr=Inherit: Same as input
  Mux1 : Mux  Inputs=6
  Product4 : Product  Inputs=3  SaturateOnIntegerOverflow=on  InputSameDT=on  OutDataTypeStr=Inherit: Same as first input
  Selector1 : Selector  InputPortWidth=4  IndexOptions=Index vector (dialog)  Indices=1  OutputSizes=1
  Sum1 : Sum  SaturateOnIntegerOverflow=on
  delCoeff : Outport
  wires:
  Actuators/1 -> Selector1/1
  Constant1/1 -> Mux1/6, Mux1/4, Mux1/2, Mux1/1
  Selector1/1 -> Product4/3, Gain1/1, Gain3/1
  Mux1/1 -> delCoeff/1
  Beta/1 -> Product4/1, Product4/2
  Product4/1 -> Gain2/1
  Sum1/1 -> Mux1/3
  Gain2/1 -> Sum1/1
  Gain1/1 -> Sum1/2
  Gain3/1 -> Mux1/5

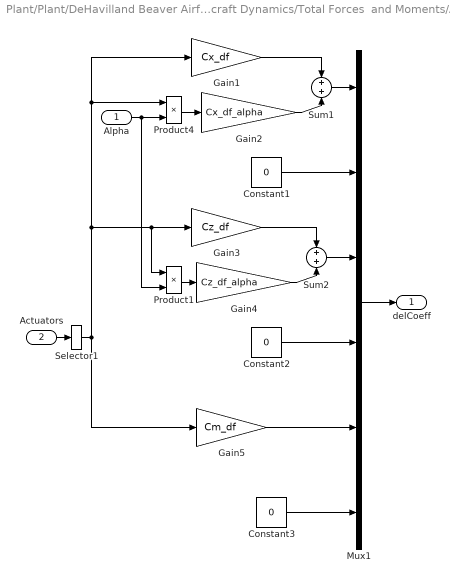
== system Plant/Plant/DeHavilland Beaver Airframe/Aircraft Dynamics/Total Forces  and Moments/Aerodynamics/Actuator Increments/Flap ==
  Alpha : Inport
  Actuators : Inport  Port=2
  Constant1 : Constant  Value=0
  Constant2 : Constant  Value=0
  Constant3 : Constant  Value=0
  Gain1 : Gain  Gain=Cx_df  SaturateOnIntegerOverflow=on  OutDataTypeStr=Inherit: Same as input  ParamDataTypeStr=Inherit: Same as input
  Gain2 : Gain  Gain=Cx_df_alpha  SaturateOnIntegerOverflow=on  OutDataTypeStr=Inherit: Same as input  ParamDataTypeStr=Inherit: Same as input
  Gain3 : Gain  Gain=Cz_df  SaturateOnIntegerOverflow=on  OutDataTypeStr=Inherit: Same as input  ParamDataTypeStr=Inherit: Same as input
  Gain4 : Gain  Gain=Cz_df_alpha  SaturateOnIntegerOverflow=on  OutDataTypeStr=Inherit: Same as input  ParamDataTypeStr=Inherit: Same as input
  Gain5 : Gain  Gain=Cm_df  SaturateOnIntegerOverflow=on  OutDataTypeStr=Inherit: Same as input  ParamDataTypeStr=Inherit: Same as input
  Mux1 : Mux  Inputs=6
  Product1 : Product  SaturateOnIntegerOverflow=on  InputSameDT=on  OutDataTypeStr=Inherit: Same as first input
  Product4 : Product  SaturateOnIntegerOverflow=on  InputSameDT=on  OutDataTypeStr=Inherit: Same as first input
  Selector1 : Selector  InputPortWidth=4  IndexOptions=Index vector (dialog)  Indices=4  OutputSizes=1
  Sum1 : Sum  SaturateOnIntegerOverflow=on
  Sum2 : Sum  SaturateOnIntegerOverflow=on
  delCoeff : Outport
  wires:
  Constant3/1 -> Mux1/6
  Constant2/1 -> Mux1/4
  Constant1/1 -> Mux1/2
  Sum2/1 -> Mux1/3
  Sum1/1 -> Mux1/1
  Mux1/1 -> delCoeff/1
  Alpha/1 -> Product4/2, Product1/2
  Product4/1 -> Gain2/1
  Gain2/1 -> Sum1/2
  Gain1/1 -> Sum1/1
  Product1/1 -> Gain4/1
  Gain4/1 -> Sum2/2
  Gain3/1 -> Sum2/1
  Gain5/1 -> Mux1/5
  Actuators/1 -> Selector1/1
  Selector1/1 -> Gain5/1, Gain3/1, Product1/1, Product4/1, Gain1/1

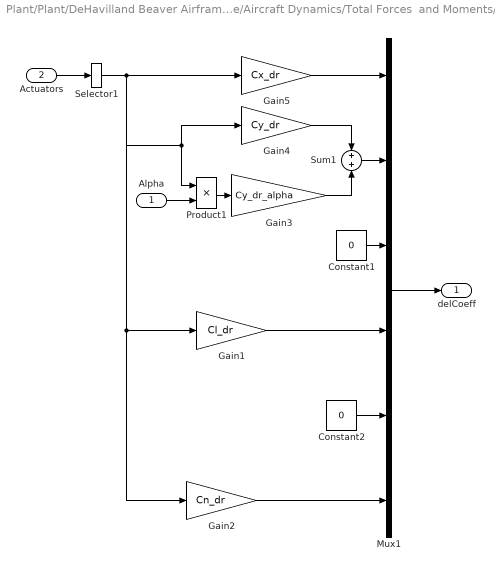
== system Plant/Plant/DeHavilland Beaver Airframe/Aircraft Dynamics/Total Forces  and Moments/Aerodynamics/Actuator Increments/Rudder ==
  Alpha : Inport
  Actuators : Inport  Port=2
  Constant1 : Constant  Value=0
  Constant2 : Constant  Value=0
  Gain1 : Gain  Gain=Cl_dr  SaturateOnIntegerOverflow=on  OutDataTypeStr=Inherit: Same as input  ParamDataTypeStr=Inherit: Same as input
  Gain2 : Gain  Gain=Cn_dr  SaturateOnIntegerOverflow=on  OutDataTypeStr=Inherit: Same as input  ParamDataTypeStr=Inherit: Same as input
  Gain3 : Gain  Gain=Cy_dr_alpha  SaturateOnIntegerOverflow=on  OutDataTypeStr=Inherit: Same as input  ParamDataTypeStr=Inherit: Same as input
  Gain4 : Gain  Gain=Cy_dr  SaturateOnIntegerOverflow=on  OutDataTypeStr=Inherit: Same as input  ParamDataTypeStr=Inherit: Same as input
  Gain5 : Gain  Gain=Cx_dr  SaturateOnIntegerOverflow=on  OutDataTypeStr=Inherit: Same as input  ParamDataTypeStr=Inherit: Same as input
  Mux1 : Mux  Inputs=6
  Product1 : Product  SaturateOnIntegerOverflow=on  InputSameDT=on  OutDataTypeStr=Inherit: Same as first input
  Selector1 : Selector  InputPortWidth=4  IndexOptions=Index vector (dialog)  Indices=3  OutputSizes=1
  Sum1 : Sum  SaturateOnIntegerOverflow=on
  delCoeff : Outport
  wires:
  Selector1/1 -> Product1/1, Gain2/1, Gain1/1, Gain4/1, Gain5/1
  Constant2/1 -> Mux1/5
  Constant1/1 -> Mux1/3
  Sum1/1 -> Mux1/2
  Actuators/1 -> Selector1/1
  Mux1/1 -> delCoeff/1
  Alpha/1 -> Product1/2
  Product1/1 -> Gain3/1
  Gain2/1 -> Mux1/6
  Gain1/1 -> Mux1/4
  Gain3/1 -> Sum1/2
  Gain4/1 -> Sum1/1
  Gain5/1 -> Mux1/1

== system Plant/Plant/DeHavilland Beaver Airframe/Aircraft Dynamics/Total Forces  and Moments/Aerodynamics/Body Rate Damping/p ==
  Constant1 : Constant  Value=0
  Constant2 : Constant  Value=Cy_p
  Constant3 : Constant  Value=Cl_p
  Constant4 : Constant  Value=Cn_p
  Mux1 : Mux  Inputs=6
  delCoeff : Outport
  wires:
  Constant3/1 -> Mux1/4
  Constant4/1 -> Mux1/6
  Constant1/1 -> Mux1/1, Mux1/3, Mux1/5
  Mux1/1 -> delCoeff/1
  Constant2/1 -> Mux1/2

== system Plant/Plant/DeHavilland Beaver Airframe/Aircraft Dynamics/Total Forces  and Moments/Aerodynamics/Body Rate Damping/q ==
  Constant1 : Constant  Value=0
  Constant2 : Constant  Value=Cz_q
  Constant3 : Constant  Value=Cx_q
  Constant4 : Constant  Value=Cm_q
  Constant5 : Constant  Value=Cn_q
  Mux1 : Mux  Inputs=6
  delCoeff : Outport
  wires:
  Mux1/1 -> delCoeff/1
  Constant3/1 -> Mux1/1
  Constant4/1 -> Mux1/5
  Constant1/1 -> Mux1/2, Mux1/4
  Constant5/1 -> Mux1/6
  Constant2/1 -> Mux1/3

== system Plant/Plant/DeHavilland Beaver Airframe/Aircraft Dynamics/Total Forces  and Moments/Aerodynamics/Body Rate Damping/r ==
  Constant : Constant  Value=0
  Constant1 : Constant  Value=Cy_r
  Constant2 : Constant  Value=Cl_r
  Constant3 : Constant  Value=Cm_r
  Constant4 : Constant  Value=Cn_r
  Mux1 : Mux  Inputs=6
  delCoeff : Outport
  wires:
  Mux1/1 -> delCoeff/1
  Constant/1 -> Mux1/1, Mux1/3
  Constant2/1 -> Mux1/4
  Constant4/1 -> Mux1/6
  Constant1/1 -> Mux1/2
  Constant3/1 -> Mux1/5
